simulink model "mElegooArduinoV1"  (R2022b)
settings: Solver=FixedStepDiscrete  StartTime=0.0  StopTime=inf  FixedStep=0.1  RelTol=1e-3  EnableMultiTasking=on
libraries: simulink x14, arduinolib x11, arduinosensorlib x1
settings Model: FPTRunName=Active  ExtModeTrigDuration=2  Creator=The MathWorks, Inc.  LastModifiedBy=ivang
settings SolverCC: AlgebraicLoopSolver=TrustRegion
settings DataIOCC: LimitDataPoints=on  ReturnWorkspaceOutputs=off
settings OptimizationCC: ExpressionDepthLimit=2147483647  LifeSpan=Inf  MaxStackSize=64
settings DebuggingCC: MergeDetectMultiDrivingBlocksExec=none  FcnCallInpInsideContextMsg=warning  UnconnectedInputMsg=warning  UnconnectedOutputMsg=warning  UnconnectedLineMsg=warning  AllowSymbolicDim=off  StateNameClashWarn=warning  SFUnexpectedBacktrackingDiag=warning  SFNoUnconditionalDefaultTransitionDiag=warning  SFExecutionAtInitializationDiag=none  SFMachineParentedDataDiag=warning  ArithmeticOperatorsInVariantConditions=warning
settings HardwareCC: ProdBitPerInt=16  ProdBitPerPointer=16  ProdBitPerSizeT=16  ProdBitPerPtrDiffT=16  ProdLargestAtomicFloat=None  ProdWordSize=8  ProdHWDeviceType=Atmel->AVR
settings ModelReferenceCC: EnableRefExpFcnMdlSchedulingChecks=on  PropagateSignalLabelsOutOfModel=off
settings SFSimCC: SimUseLocalCustomCode=off  MATLABDynamicMemAlloc=off
settings RTWCC: Description=Embedded Coder  SystemTargetFile=ert.tlc  HardwareBoard=Arduino Uno  TemplateMakefile=ert_default_tmf  GenerateReport=on  RTWVerbose=off  RTWUseLocalCustomCode=off  Toolchain=Arduino AVR  BuildConfiguration=Faster Runs  LaunchReport=on  DLArmComputeVersion=19.05
settings CodeAppCC: ForceParamTrailComments=on  OperatorAnnotations=on  StateflowObjectComments=on  MATLABSourceComments=on
settings ERTTargetCC: MultiwordLength=2048  ERTCustomFileBanners=off  SupportContinuousTime=on  SupportNonInlinedSFcns=on  RemoveResetFunc=off  SupportVariableSizeSignals=on  ModelStepFunctionPrototypeControlCompliant=off  ExtModeTransport=3  ExtModeStaticAlloc=on  ExtModeAutomaticAllocSize=off  ExtModeStaticAllocSize=250  ExtModeMexFile=ext_xcp  ExtModeIntrfLevel=Level2 - Open
settings ConfigComp: CovMetricSettings=dw  CovSaveCumulativeToWorkspaceVar=on  CovSaveSingleToWorkspaceVar=on  CovExternalEMLEnable=off  CovSFcnEnable=off

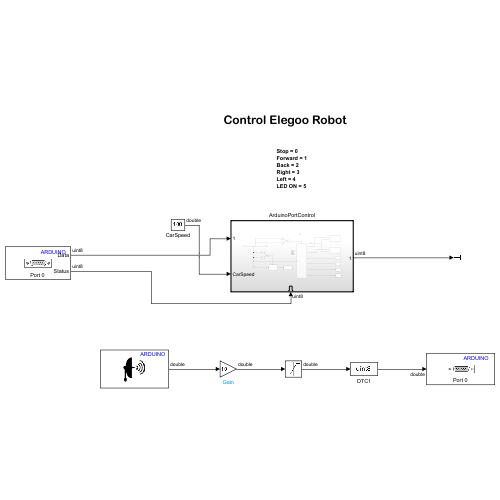
[thumbnail: Simulink's stored preview of the top-level diagram]
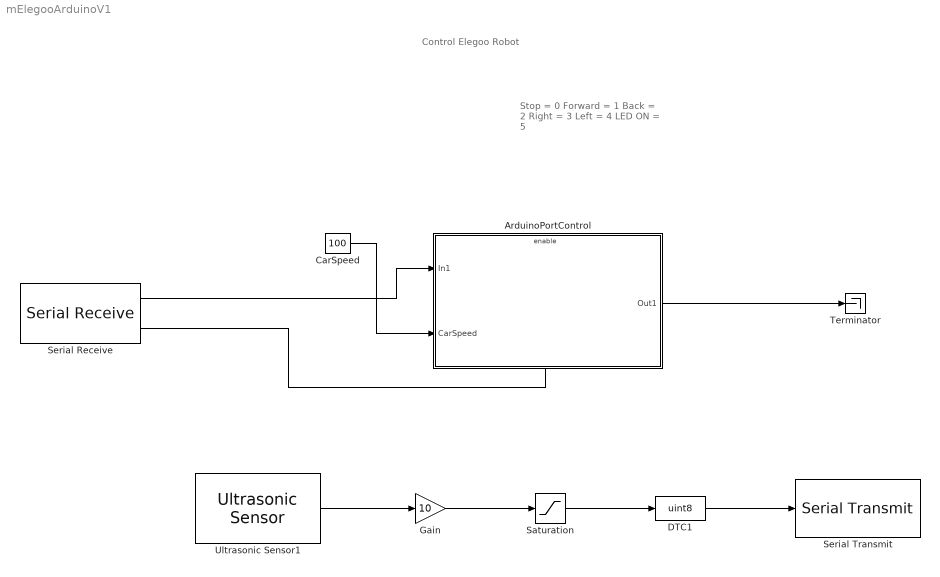
== system mElegooArduinoV1 ==
  note: Control Elegoo Robot
  note: Stop = 0
      | Forward = 1
      | Back = 2
      | Right = 3
      | Left = 4
      | LED ON = 5
  ArduinoPortControl : Subsystem
  CarSpeed : Constant  Value=100
  DTC1 : DataTypeConversion  OutDataTypeStr=uint8  SaturateOnIntegerOverflow=off  RndMeth=Floor
  Gain : Gain  Gain=10  OutDataTypeStr=double
  Saturation : Saturate  UpperLimit=100  LowerLimit=0
  Serial Receive : arduinolib/Serial Receive  isARMArch=off  portNumber=0  DataType=uint8  Datalength=1  SampleTime=0.1  showOutStatus=on  blockPlatform=arduino
  Serial Transmit : arduinolib/Serial Transmit  portNumber=0  sendmode=write  sendformat=Decimal  floatprecision=2  blockPlatform=arduino
  Terminator : Terminator
  Ultrasonic Sensor1 : arduinosensorlib/Ultrasonic Sensor  NumSignalPins=2  TrigPin=19  EchoPin=18  SignalPin=2  SampleTime_=0.1  blockPlatform=ARDUINO
  wires:
  Serial Receive/1 -> ArduinoPortControl/1(In1)
  Serial Receive/2 -> ArduinoPortControl/Enable
  CarSpeed/1 -> ArduinoPortControl/2(CarSpeed)
  ArduinoPortControl/1(Out1) -> Terminator/1
  Saturation/1 -> DTC1/1
  Ultrasonic Sensor1/1 -> Gain/1
  Gain/1 -> Saturation/1
  DTC1/1 -> Serial Transmit/1

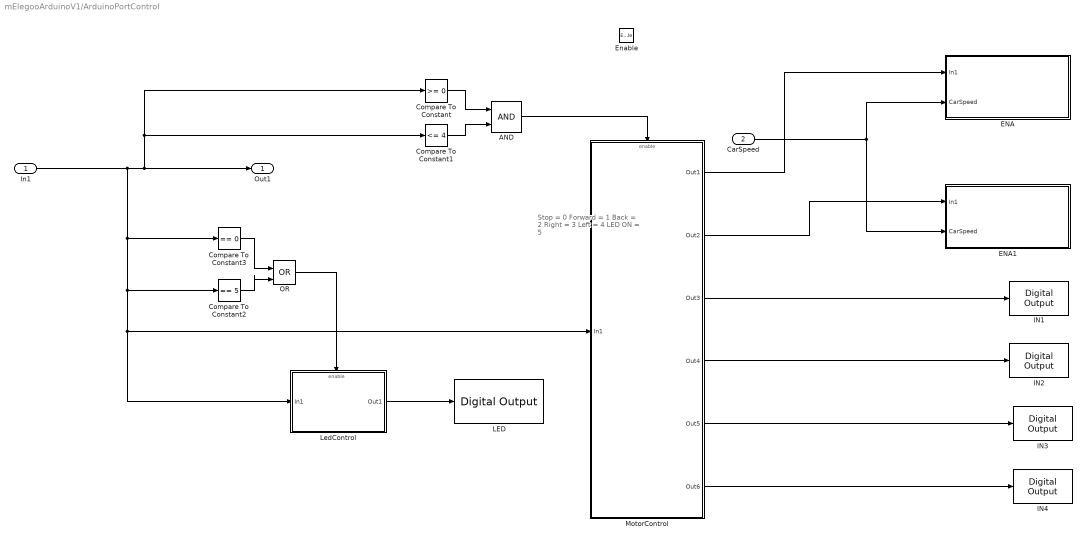
== system mElegooArduinoV1/ArduinoPortControl ==
  note: Stop = 0
      | Forward = 1
      | Back = 2
      | Right = 3
      | Left = 4
      | LED ON = 5
  In1 : Inport
  CarSpeed : Inport  Port=2
  Enable : EnablePort
  AND : Logic  IconShape=distinctive  AllPortsSameDT=off  OutDataTypeStr=boolean
  Compare To Constant : simulink/Logic and Bit Operations/Compare To Constant  relop=>=  const=0  OutDataTypeStr=boolean
  Compare To Constant1 : simulink/Logic and Bit Operations/Compare To Constant  relop=<=  const=4  OutDataTypeStr=boolean
  Compare To Constant2 : simulink/Logic and Bit Operations/Compare To Constant  relop===  const=5  OutDataTypeStr=boolean
  Compare To Constant3 : simulink/Logic and Bit Operations/Compare To Constant  relop===  const=0  OutDataTypeStr=boolean
  ENA : Subsystem  TreatAsAtomicUnit=on
  ENA1 : Subsystem  TreatAsAtomicUnit=on
  IN1 : arduinolib/Digital Output  pinNumber=6  Direction=output  blockPlatform=arduino
  IN2 : arduinolib/Digital Output  pinNumber=7  Direction=output  blockPlatform=arduino
  IN3 : arduinolib/Digital Output  pinNumber=8  Direction=output  blockPlatform=arduino
  IN4 : arduinolib/Digital Output  pinNumber=9  Direction=output  blockPlatform=arduino
  LED : arduinolib/Digital Output  pinNumber=13  Direction=output  blockPlatform=arduino
  LedControl : Subsystem
  MotorControl : Subsystem
  OR : Logic  Operator=OR  IconShape=distinctive  AllPortsSameDT=off  OutDataTypeStr=boolean
  Out1 : Outport  VectorParamsAs1DForOutWhenUnconnected=off
  wires:
  In1/1 -> LedControl/1(In1), MotorControl/1(In1), Compare To Constant2/1, Compare To Constant3/1, Compare To Constant1/1, Compare To Constant/1, Out1/1
  MotorControl/3(Out3) -> IN1/1
  MotorControl/4(Out4) -> IN2/1
  MotorControl/5(Out5) -> IN3/1
  MotorControl/6(Out6) -> IN4/1
  Compare To Constant/1 -> AND/1
  Compare To Constant1/1 -> AND/2
  AND/1 -> MotorControl/Enable
  Compare To Constant2/1 -> OR/2
  Compare To Constant3/1 -> OR/1
  LedControl/1(Out1) -> LED/1
  OR/1 -> LedControl/Enable
  MotorControl/1(Out1) -> ENA/1(In1)
  CarSpeed/1 -> ENA1/2(CarSpeed), ENA/2(CarSpeed)
  MotorControl/2(Out2) -> ENA1/1(In1)

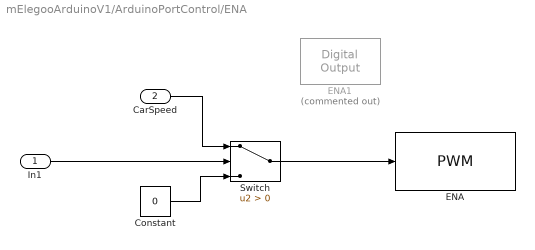
== system mElegooArduinoV1/ArduinoPortControl/ENA ==
  In1 : Inport
  CarSpeed : Inport  Port=2
  Constant : Constant  Value=0
  ENA : arduinolib/PWM  pinNumber=5  frequencyType=Default  desiredFrequency=490.2  achievableFrequency=490.2
  ENA1 : arduinolib/Digital Output  Commented=on  pinNumber=5  Direction=output  blockPlatform=arduino
  Switch : Switch  Criteria=u2 > Threshold  SaturateOnIntegerOverflow=off  InputSameDT=off
  wires:
  In1/1 -> Switch/2
  Switch/1 -> ENA/1
  Constant/1 -> Switch/3
  CarSpeed/1 -> Switch/1

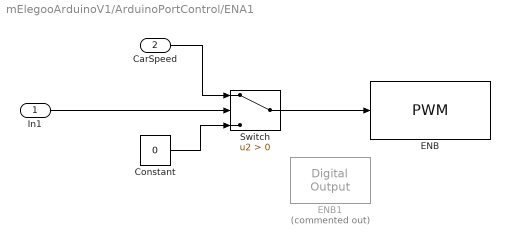
== system mElegooArduinoV1/ArduinoPortControl/ENA1 ==
  In1 : Inport
  CarSpeed : Inport  Port=2
  Constant : Constant  Value=0
  ENB : arduinolib/PWM  pinNumber=11  frequencyType=Default  desiredFrequency=490.2  achievableFrequency=490.2
  ENB1 : arduinolib/Digital Output  Commented=on  pinNumber=11  Direction=output  blockPlatform=arduino
  Switch : Switch  Criteria=u2 > Threshold  SaturateOnIntegerOverflow=off  InputSameDT=off
  wires:
  In1/1 -> Switch/2
  Switch/1 -> ENB/1
  Constant/1 -> Switch/3
  CarSpeed/1 -> Switch/1

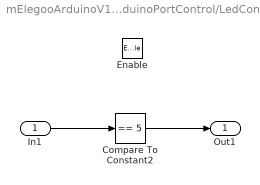
== system mElegooArduinoV1/ArduinoPortControl/LedControl ==
  In1 : Inport
  Enable : EnablePort
  Compare To Constant2 : simulink/Logic and Bit Operations/Compare To Constant  relop===  const=5  OutDataTypeStr=boolean
  Out1 : Outport
  wires:
  In1/1 -> Compare To Constant2/1
  Compare To Constant2/1 -> Out1/1

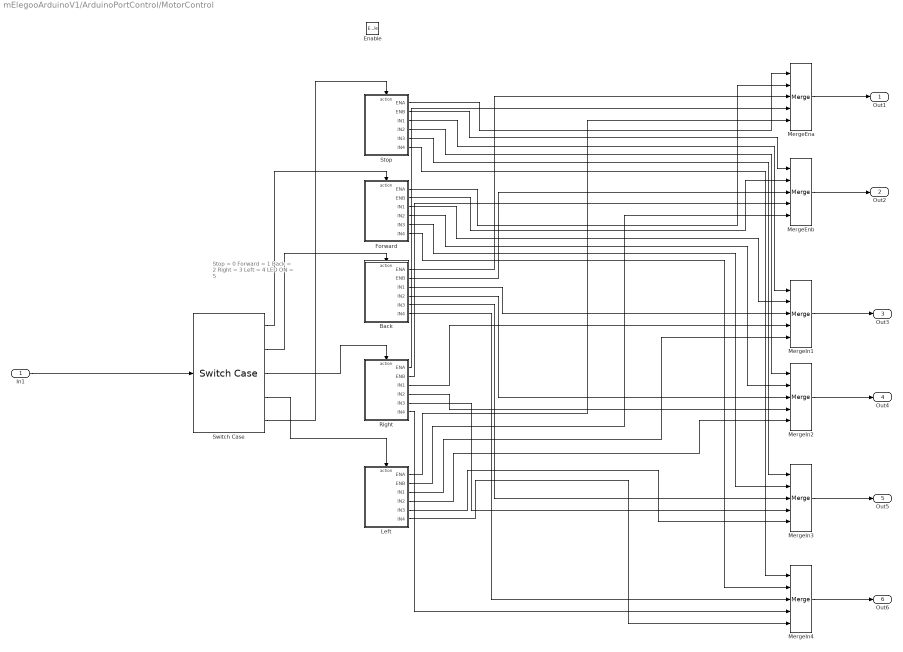
== system mElegooArduinoV1/ArduinoPortControl/MotorControl ==
  note: Stop = 0
      | Forward = 1
      | Back = 2
      | Right = 3
      | Left = 4
      | LED ON = 5
  In1 : Inport
  Enable : EnablePort
  Back : Subsystem
  Forward : Subsystem
  Left : Subsystem
  MergeEna : Merge  Inputs=5
  MergeEnb : Merge  Inputs=5
  MergeIn{1..4} (4 alike) : Merge  Inputs=5
  Right : Subsystem
  Stop : Subsystem
  Switch Case : SwitchCase  CaseConditions={1, 2, 3, 4}
  Out1 : Outport
  Out2 : Outport  Port=2
  Out3 : Outport  Port=3
  Out4 : Outport  Port=4
  Out5 : Outport  Port=5
  Out6 : Outport  Port=6
  wires:
  Left/1(ENA) -> MergeEna/5
  Switch Case/3 -> Right/Action
  Right/4(IN2) -> MergeIn2/4
  MergeEnb/1 -> Out2/1
  Stop/2(ENB) -> MergeEnb/1
  Forward/2(ENB) -> MergeEnb/2
  Back/2(ENB) -> MergeEnb/3
  In1/1 -> Switch Case/1
  Switch Case/2 -> Back/Action
  Forward/4(IN2) -> MergeIn2/2
  Back/3(IN1) -> MergeIn1/3
  Forward/5(IN3) -> MergeIn3/2
  Back/6(IN4) -> MergeIn4/3
  Left/3(IN1) -> MergeIn1/5
  Stop/4(IN2) -> MergeIn2/1
  Right/1(ENA) -> MergeEna/4
  Forward/1(ENA) -> MergeEna/2
  Back/5(IN3) -> MergeIn3/3
  Switch Case/5 -> Stop/Action
  Stop/5(IN3) -> MergeIn3/1
  Switch Case/4 -> Left/Action
  Left/2(ENB) -> MergeEnb/5
  Stop/6(IN4) -> MergeIn4/1
  MergeIn4/1 -> Out6/1
  Back/1(ENA) -> MergeEna/3
  MergeIn2/1 -> Out4/1
  Back/4(IN2) -> MergeIn2/3
  Right/2(ENB) -> MergeEnb/4
  Forward/3(IN1) -> MergeIn1/2
  Switch Case/1 -> Forward/Action
  MergeEna/1 -> Out1/1
  Left/4(IN2) -> MergeIn2/5
  MergeIn1/1 -> Out3/1
  Stop/3(IN1) -> MergeIn1/1
  Right/3(IN1) -> MergeIn1/4
  MergeIn3/1 -> Out5/1
  Forward/6(IN4) -> MergeIn4/2
  Stop/1(ENA) -> MergeEna/1
  Right/5(IN3) -> MergeIn3/4
  Left/5(IN3) -> MergeIn3/5
  Right/6(IN4) -> MergeIn4/4
  Left/6(IN4) -> MergeIn4/5

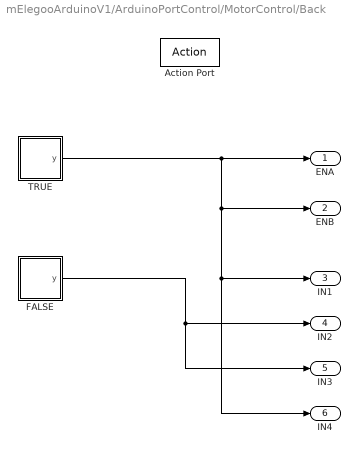
== system mElegooArduinoV1/ArduinoPortControl/MotorControl/Back ==
  Action Port : ActionPort  ActionPortLabel=case [ 2 ]:
  FALSE : Subsystem
  TRUE : Subsystem
  ENA : Outport
  ENB : Outport  Port=2
  IN1 : Outport  Port=3
  IN2 : Outport  Port=4
  IN3 : Outport  Port=5
  IN4 : Outport  Port=6
  wires:
  TRUE/1(y) -> IN4/1, IN1/1, ENB/1, ENA/1
  FALSE/1(y) -> IN3/1, IN2/1

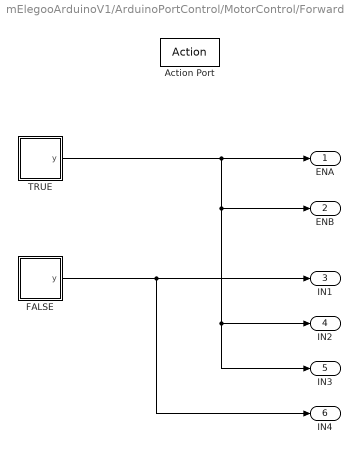
== system mElegooArduinoV1/ArduinoPortControl/MotorControl/Forward ==
  Action Port : ActionPort  ActionPortLabel=case [ 1 ]:
  FALSE : Subsystem
  TRUE : Subsystem
  ENA : Outport
  ENB : Outport  Port=2
  IN1 : Outport  Port=3
  IN2 : Outport  Port=4
  IN3 : Outport  Port=5
  IN4 : Outport  Port=6
  wires:
  FALSE/1(y) -> IN4/1, IN1/1
  TRUE/1(y) -> IN3/1, IN2/1, ENB/1, ENA/1

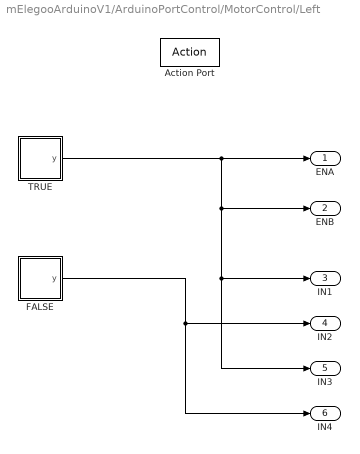
== system mElegooArduinoV1/ArduinoPortControl/MotorControl/Left ==
  Action Port : ActionPort  ActionPortLabel=case [ 4 ]:
  FALSE : Subsystem
  TRUE : Subsystem
  ENA : Outport
  ENB : Outport  Port=2
  IN1 : Outport  Port=3
  IN2 : Outport  Port=4
  IN3 : Outport  Port=5
  IN4 : Outport  Port=6
  wires:
  TRUE/1(y) -> IN3/1, IN1/1, ENB/1, ENA/1
  FALSE/1(y) -> IN4/1, IN2/1

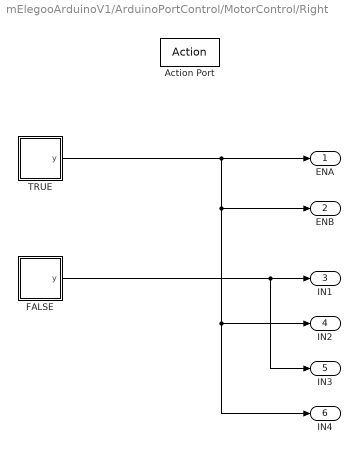
== system mElegooArduinoV1/ArduinoPortControl/MotorControl/Right ==
  Action Port : ActionPort  ActionPortLabel=case [ 3 ]:
  FALSE : Subsystem
  TRUE : Subsystem
  ENA : Outport
  ENB : Outport  Port=2
  IN1 : Outport  Port=3
  IN2 : Outport  Port=4
  IN3 : Outport  Port=5
  IN4 : Outport  Port=6
  wires:
  TRUE/1(y) -> IN4/1, IN2/1, ENB/1, ENA/1
  FALSE/1(y) -> IN3/1, IN1/1

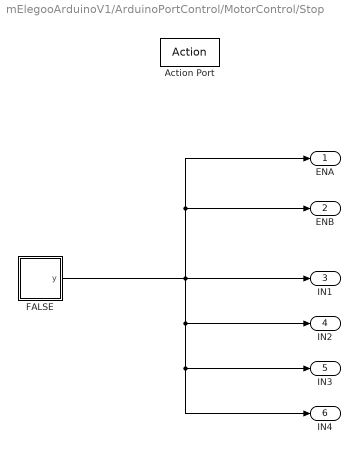
== system mElegooArduinoV1/ArduinoPortControl/MotorControl/Stop ==
  Action Port : ActionPort  ActionPortLabel=default:
  FALSE : Subsystem
  ENA : Outport
  ENB : Outport  Port=2
  IN1 : Outport  Port=3
  IN2 : Outport  Port=4
  IN3 : Outport  Port=5
  IN4 : Outport  Port=6
  wires:
  FALSE/1(y) -> IN1/1, IN2/1, IN3/1, IN4/1, ENB/1, ENA/1

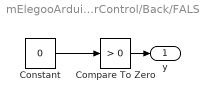
== system mElegooArduinoV1/ArduinoPortControl/MotorControl/Back/FALSE ==
  Compare To Zero : simulink/Logic and Bit Operations/Compare To Zero  relop=>  OutDataTypeStr=boolean
  Constant : Constant  Value=0
  y : Outport
  wires:
  Constant/1 -> Compare To Zero/1
  Compare To Zero/1 -> y/1

== system mElegooArduinoV1/ArduinoPortControl/MotorControl/Back/TRUE ==
  Compare To Zero : simulink/Logic and Bit Operations/Compare To Zero  relop=>  OutDataTypeStr=boolean
  Constant : Constant
  y : Outport
  wires:
  Constant/1 -> Compare To Zero/1
  Compare To Zero/1 -> y/1

== system mElegooArduinoV1/ArduinoPortControl/MotorControl/Forward/FALSE ==
  Compare To Zero : simulink/Logic and Bit Operations/Compare To Zero  relop=>  OutDataTypeStr=boolean
  Constant : Constant  Value=0
  y : Outport
  wires:
  Constant/1 -> Compare To Zero/1
  Compare To Zero/1 -> y/1

== system mElegooArduinoV1/ArduinoPortControl/MotorControl/Forward/TRUE ==
  Compare To Zero : simulink/Logic and Bit Operations/Compare To Zero  relop=>  OutDataTypeStr=boolean
  Constant : Constant
  y : Outport
  wires:
  Constant/1 -> Compare To Zero/1
  Compare To Zero/1 -> y/1

== system mElegooArduinoV1/ArduinoPortControl/MotorControl/Left/FALSE ==
  Compare To Zero : simulink/Logic and Bit Operations/Compare To Zero  relop=>  OutDataTypeStr=boolean
  Constant : Constant  Value=0
  y : Outport
  wires:
  Constant/1 -> Compare To Zero/1
  Compare To Zero/1 -> y/1

== system mElegooArduinoV1/ArduinoPortControl/MotorControl/Left/TRUE ==
  Compare To Zero : simulink/Logic and Bit Operations/Compare To Zero  relop=>  OutDataTypeStr=boolean
  Constant : Constant
  y : Outport
  wires:
  Constant/1 -> Compare To Zero/1
  Compare To Zero/1 -> y/1

== system mElegooArduinoV1/ArduinoPortControl/MotorControl/Right/FALSE ==
  Compare To Zero : simulink/Logic and Bit Operations/Compare To Zero  relop=>  OutDataTypeStr=boolean
  Constant : Constant  Value=0
  y : Outport
  wires:
  Constant/1 -> Compare To Zero/1
  Compare To Zero/1 -> y/1

== system mElegooArduinoV1/ArduinoPortControl/MotorControl/Right/TRUE ==
  Compare To Zero : simulink/Logic and Bit Operations/Compare To Zero  relop=>  OutDataTypeStr=boolean
  Constant : Constant
  y : Outport
  wires:
  Constant/1 -> Compare To Zero/1
  Compare To Zero/1 -> y/1

== system mElegooArduinoV1/ArduinoPortControl/MotorControl/Stop/FALSE ==
  Compare To Zero : simulink/Logic and Bit Operations/Compare To Zero  relop=>  OutDataTypeStr=boolean
  Constant : Constant  Value=0
  y : Outport
  wires:
  Constant/1 -> Compare To Zero/1
  Compare To Zero/1 -> y/1
